simulink model "EjercicioControl"  (R2020b)
settings: Solver=FixedStepAuto  StartTime=0.0  StopTime=100  FixedStep=0.02  RelTol=1e-3
values from neighbouring files (symbols this model uses):
  I = RGB    [imagesGeneration.m]    (also in modifierSize.m)
undefined symbols (not defined in the file or in its folder): F
libraries: androiduilib x8, pid_lib x1, androidaudiovideolib x1
settings Model: Creator=earui  LastModifiedBy=earui
settings OptimizationCC: EnhancedBackFolding=on  PassReuseOutputArgsAs=Individual arguments  ZeroExternalMemoryAtStartup=off  ZeroInternalMemoryAtStartup=off  MaxStackSize=64  OptimizeBlockOrder=speed  DifferentSizesBufferReuse=on  OptimizationCustomize=off  EfficientTunableParamExpr=on
settings DebuggingCC: ParameterTunabilityLossMsg=error
settings HardwareCC: ProdBitPerPointer=32  ProdBitPerSizeT=32  ProdBitPerPtrDiffT=32  ProdLargestAtomicInteger=Long  ProdLargestAtomicFloat=Double  ProdWordSize=32  ProdHWDeviceType=ARM Compatible->ARM Cortex
settings SFSimCC: MATLABDynamicMemAlloc=off
settings RTWCC: Description=Embedded Coder  SystemTargetFile=ert.tlc  HardwareBoard=Android Device  TLCOptions="-aInlineSetEventsForThisBaseRateFcn=TLC_FALSE -aSuppressMultiTaskScheduler=TLC_FALSE  -aRateBasedStepFcn=0"  TemplateMakefile=ert_default_tmf  RTWVerbose=off  Toolchain=Android SDK/NDK Tools
settings CodeAppCC: ForceParamTrailComments=on  IgnoreCustomStorageClasses=off  OperatorAnnotations=on  SimulinkDataObjDesc=on  SFDataObjDesc=on  InsertBlockDesc=on
settings ERTTargetCC: SupportContinuousTime=on

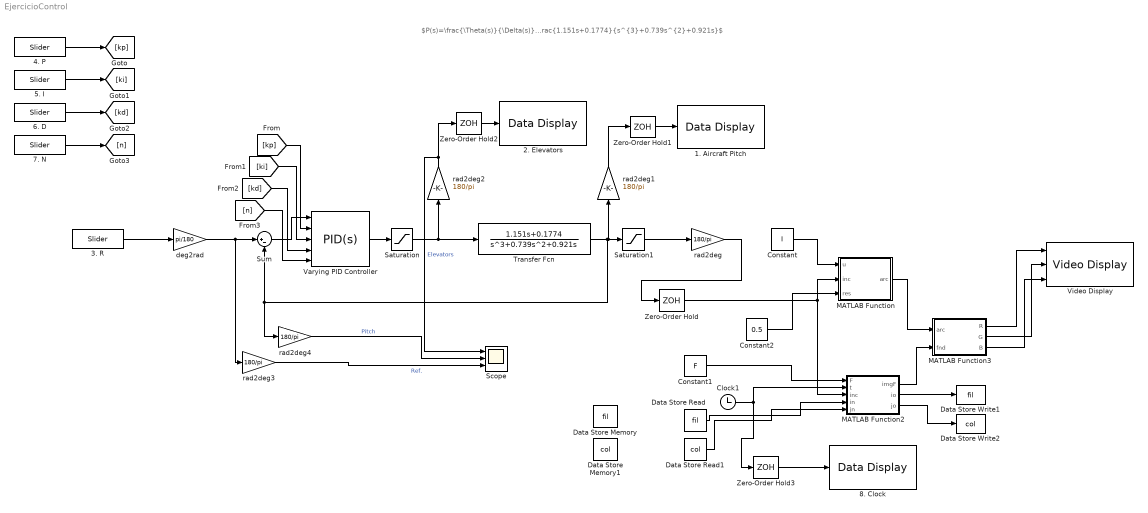
== system EjercicioControl ==
  note: $P(s)=\frac{\Theta(s)}{\Delta(s)}=\frac{1.151s+0.1774}{s^{3}+0.739s^{2}+0.921s}$
  1. Aircraft Pitch : androiduilib/Data Display  DataDisplayId=EjercicioControl/1._Aircraft_Pitch  Format=Float  Precision=1  SimulateUsing=Code generation  blockPlatform=Android
      settings: SourceProductBaseCode=ANDROID
  2. Elevators : androiduilib/Data Display  DataDisplayId=EjercicioControl/2._Elevators  Format=Float  Precision=2  SimulateUsing=Code generation  blockPlatform=Android
      settings: SourceProductBaseCode=ANDROID
  3. R : androiduilib/Slider  Min=-30  Value=0  Max=30  Resolution=1  SliderId=EjercicioControl/3._R  SampleTime=0.04  BlockPlatform=Android
      settings: SourceProductBaseCode=ANDROID
  4. P : androiduilib/Slider  Min=0  Value=10  Max=75  Resolution=0.25  SliderId=EjercicioControl/4._P  SampleTime=0.04  BlockPlatform=Android
      settings: SourceProductBaseCode=ANDROID
  5. I : androiduilib/Slider  Min=0  Value=1  Max=25  Resolution=0.25  SliderId=EjercicioControl/5._I  SampleTime=0.04  BlockPlatform=Android
      settings: SourceProductBaseCode=ANDROID
  6. D : androiduilib/Slider  Min=0  Value=1  Max=25  Resolution=0.25  SliderId=EjercicioControl/6._D  SampleTime=0.04  BlockPlatform=Android
      settings: SourceProductBaseCode=ANDROID
  7. N : androiduilib/Slider  Min=0  Value=100  Max=200  Resolution=10  SliderId=EjercicioControl/7._N  SampleTime=0.04  BlockPlatform=Android
      settings: SourceProductBaseCode=ANDROID
  8. Clock : androiduilib/Data Display  DataDisplayId=EjercicioControl/8._Clock  Format=Float  Precision=1  SimulateUsing=Code generation  blockPlatform=Android
      settings: SourceProductBaseCode=ANDROID
  Clock1 : Clock
      settings: Decimation=3
  Constant : Constant  Value=I
  Constant1 : Constant  Value=F
  Constant2 : Constant  Value=0.5
  Data Store Memory : DataStoreMemory  DataStoreName=fil  ReadBeforeWriteMsg=warning  WriteAfterWriteMsg=warning  WriteAfterReadMsg=warning  ShowAdditionalParam=off
  Data Store Memory1 : DataStoreMemory  DataStoreName=col  ReadBeforeWriteMsg=warning  WriteAfterWriteMsg=warning  WriteAfterReadMsg=warning  ShowAdditionalParam=off
  Data Store Read : DataStoreRead  DataStoreName=fil
  Data Store Read1 : DataStoreRead  DataStoreName=col
  Data Store Write1 : DataStoreWrite  DataStoreName=fil
  Data Store Write2 : DataStoreWrite  DataStoreName=col
  MATLAB Function : MATLAB Function  TreatAsAtomicUnit=on
  MATLAB Function2 : MATLAB Function  TreatAsAtomicUnit=on
  MATLAB Function3 : MATLAB Function  TreatAsAtomicUnit=on
  Saturation : Saturate  UpperLimit=2*pi/9  LowerLimit=-2*pi/9
  Saturation1 : Saturate  UpperLimit=pi/4  LowerLimit=-pi/4
  Scope : Scope  NumInputPorts=3
  Sum : Sum  Inputs=|+-
  Transfer Fcn : TransferFcn  Numerator=[1.151 0.1774]  Denominator=[1 0.739 0.921 0]
  Varying PID Controller : pid_lib/PID Controller  Controller=PID  Form=Parallel  TimeDomain=Continuous-time  UseExternalTs=off  SampleTime=-1  IntegratorMethod=Forward Euler  FilterMethod=Forward Euler  ControllerParametersSource=external  P=1  I=1  D=0  UseFilter=on  N=100  TunerSelectOption=Transfer Function Based (PID Tuner App)  InitialConditionSource=internal  InitialConditionForIntegrator=0  InitialConditionForFilter=0  DifferentiatorICPrevScaledInput=0  ExternalReset=none  TrackingMode=off  Kt=1  LimitOutput=off  SatLimitsSource=internal  UpperSaturationLimit=inf  LowerSaturationLimit=-inf  LinearizeAsGain=on  AntiWindupMode=none  Kb=1  POutMin=[]  POutMax=[]  IOutMin=[]  IOutMax=[]  DOutMin=[]  DOutMax=[]  NOutMin=[]  NOutMax=[]  SumOutMin=[]  SumOutMax=[]  SaturationOutMin=[]  SaturationOutMax=[]  PParamMin=[]  PParamMax=[]  IParamMin=[]  IParamMax=[]  DParamMin=[]  DParamMax=[]  NParamMin=[]  NParamMax=[]  KbParamMin=[]  KbParamMax=[]  KtParamMin=[]  KtParamMax=[]  KbOutMin=[]  KbOutMax=[]  KtOutMin=[]  KtOutMax=[]  IntegratorOutMin=[]  IntegratorOutMax=[]  FilterOutMin=[]  FilterOutMax=[]  SumI1OutMin=[]  SumI1OutMax=[]  SumI2OutMin=[]  SumI2OutMax=[]  SumI3OutMin=[]  SumI3OutMax=[]  SumI4OutMin=[]  SumI4OutMax=[]  SumDOutMin=[]  SumDOutMax=[]  DifferentiatorOutMin=[]  DifferentiatorOutMax=[]  FilterDiffOutCoefMin=[]  FilterDiffOutCoefMax=[]  ReciprocalOutMin=[]  ReciprocalOutMax=[]  SumDenOutMin=[]  SumDenOutMax=[]  SumNumOutMin=[]  SumNumOutMax=[]  DivideOutMin=[]  DivideOutMax=[]  UdiffTsProdOutMin=[]  UdiffTsProdOutMax=[]  NTsProdOutMin=[]  NTsProdOutMax=[]  UintegralTsProdOutMin=[]  UintegralTsProdOutMax=[]  UngainTsProdOutMin=[]  UngainTsProdOutMax=[]  IntegratorContinuousStateAttributes=''  IntegratorStateMustResolveToSignalObject=off  IntegratorRTWStateStorageClass=Auto  FilterContinuousStateAttributes=''  FilterStateMustResolveToSignalObject=off  FilterRTWStateStorageClass=Auto  ParallelPVariant=ExternalParameters  IdealPVariant=Disabled  IVariant=ExternalParameters  DVariant=ExternalParameters  IntegratorVariant=Continuous  SatVariant=Disabled  AWVariant=Passthrough  PCopyVariant=Disabled  TRVariant=Disabled  FdbkBlocksVariant=Forward  IdealPFdbkVariant=Disabled  SatFdbkVariant=Disabled  DerivativeFilterVariant=ContFilter  NVariant=ExternalParameters  NCopyVariant=Disabled  FilterICVariant=InternalICsFilter  IntegratorICVariant=InternalICs  ExternalResetVariant=Disabled  TRSumVariant=Passthrough  SumFdbkVariant=Disabled  SumVariant=Sum_PID  TsampFilterVariant=InternalTs  TsampNgainVariant=Passthrough  TsampIntegralVariant=Passthrough  ExternalSaturationOutDataTypeStr=Inherit: Same as second input
  Video Display : androidaudiovideolib/Video Display  BlockPlatform=Android
      settings: SourceProductBaseCode=ANDROID
  Zero-Order Hold : ZeroOrderHold  SampleTime=0.04
  Zero-Order Hold1 : ZeroOrderHold  SampleTime=0.1
  Zero-Order Hold2 : ZeroOrderHold  SampleTime=0.1
  Zero-Order Hold3 : ZeroOrderHold
  deg2rad : Gain  Gain=pi/180
  rad2deg{,1..4} (5 alike) : Gain  Gain=180/pi
  wires:
  Transfer Fcn/1 -> rad2deg1/1, Saturation1/1, rad2deg4/1, Sum/2
  deg2rad/1 -> rad2deg3/1, Sum/1
  Saturation/1 -> rad2deg2/1, Transfer Fcn/1
  Varying PID Controller/1 -> Saturation/1
  rad2deg/1 -> Zero-Order Hold/1
  Saturation1/1 -> rad2deg/1
  Constant/1 -> MATLAB Function/1(u)
  Zero-Order Hold/1 -> MATLAB Function2/3(inc), MATLAB Function/2(inc)
  4. P/1 -> [kp]
  Sum/1 -> Varying PID Controller/1
  [kp] -> Varying PID Controller/2
  [ki] -> Varying PID Controller/3
  [kd] -> Varying PID Controller/4
  [n] -> Varying PID Controller/5
  5. I/1 -> [ki]
  6. D/1 -> [kd]
  7. N/1 -> [n]
  3. R/1 -> deg2rad/1
  Constant1/1 -> MATLAB Function2/1(F)
  MATLAB Function2/1(imgF) -> MATLAB Function3/2(fnd)
  MATLAB Function/1(arc) -> MATLAB Function3/1(arc)
  MATLAB Function3/1(R) -> Video Display/1
  MATLAB Function3/2(G) -> Video Display/2
  MATLAB Function3/3(B) -> Video Display/3
  Constant2/1 -> MATLAB Function/3(res)
  rad2deg3/1 -> Scope/3  "Ref."
  rad2deg4/1 -> Scope/2  "Pitch"
  Clock1/1 -> Zero-Order Hold3/1, MATLAB Function2/2(t)
  Data Store Read/1 -> MATLAB Function2/4(in)
  Data Store Read1/1 -> MATLAB Function2/5(jn)
  MATLAB Function2/2(io) -> Data Store Write1/1
  MATLAB Function2/3(jo) -> Data Store Write2/1
  rad2deg2/1 -> Scope/1, Zero-Order Hold2/1  "Elevators"
  Zero-Order Hold2/1 -> 2. Elevators/1
  rad2deg1/1 -> Zero-Order Hold1/1
  Zero-Order Hold1/1 -> 1. Aircraft Pitch/1
  Zero-Order Hold3/1 -> 8. Clock/1

== matlab function EjercicioControl/MATLAB Function ==
  data: u input; arc output; inc input; res input
function arc   = fcn(u,inc,res)
ind=round((inc+45)/res)+1;
R=u(:,:,1,ind);
G=u(:,:,2,ind);
B=u(:,:,3,ind);

arc = cat(3,R,G,B);

end

== matlab function EjercicioControl/MATLAB Function2 ==
  data: imgF output; F input; t input; inc input; in input; jn input; io output; jo output
function [imgF, io, jo]  = fcn(F,t,inc, in, jn) %, jO |   , jI
tAux=t*1000;

if  mod(tAux,20)==0
    if inc>=-60 && inc<-46
        io=in+3;
        jo=jn-4;
    elseif inc>=-46 && inc<-30.5
        io=in+4;
        jo=jn-3;
    elseif inc>=-30.5 && inc<-17.5
        io=in+5;
        jo=jn-2;
    elseif inc>=-17.5 && inc<-6
        io=in+5;
        jo=jn-1;
        
    elseif inc>=-6 && inc<=6
        io=in+5;
        jo=jn;
        
    elseif inc>6 && inc<=17.5
        io=in+5;
        jo=jn+1;
    elseif inc>17.5 && inc<=30.5
        io=in+5;
        jo=jn+2;  
    elseif inc>30.5 && inc<=46
        io=in+4;
        jo=jn+3;
    else
        io=in+3;
        jo=jn+4;
    end
else
    io=in;
    jo=jn;
end
imgF=circshift(F,[io jo]);

    



% if inc<=8 && inc>=-8
%     jO=jI;
% elseif inc<=30 && inc>8
%         if  mod(tAux,16)==0
%             jO=jI+1;
%         else
%             jO=jI;
%         end
% elseif inc>30 || inc<-8
%         if  mod(tAux,16)==0
%             jO=jI-1;
%         else
%             jO=jI;
%         end
% else
%         imgF=F;
%         jO=jI;
% end

== matlab function EjercicioControl/MATLAB Function3 ==
  data: arc input; R output; fnd input; G output; B output
function [R, G, B] = fcn(arc, fnd)
R=arc(:,:,1);
G=arc(:,:,2);
B=arc(:,:,3);
Rf=fnd(:,:,1);
Gf=fnd(:,:,2);
Bf=fnd(:,:,3);
for i=1:527
    for j=1:527
        if R(i,j)<=25 && G(i,j)<=25 && B(i,j)<=25
            R(i,j)=Rf(i,j);
            G(i,j)=Gf(i,j);
            B(i,j)=Bf(i,j);
        else
            R(i,j)=R(i,j);
            G(i,j)=G(i,j);
            B(i,j)=B(i,j);
        end
    end
end
